simulink model "actuator_control"  (R2015a)
settings: Solver=FixedStepDiscrete  StartTime=0.0  StopTime=inf  FixedStep=sample_time  RelTol=1e-3
undefined symbols (not defined in the file): A_kalman_swing_load, A_lpf_dtau, B1_lpf_dtau, B2_lpf_dtau, B_kalman_swing_load, C_kalman_swing_load, Discrete, fdesignblkfcn, gcbh, initial_dx_estimate, j_segments, k_sea_low, lateral_motor_efficiency, P0_kalman_swing_load, sample_time, swing_collision_damping_rate, Time
libraries: simulink x11, dsparch4 x6, ctrlSharedLib x4, dspfdesign x2
(part 1 of 2)
settings Model: CovSFcnEnable=off  Creator=wmartin  LastModifiedBy=wmartin
settings SolverCC: EnableConcurrentExecution=on
settings DataIOCC: MaxDataPoints=1000000000  SaveFormat=StructureWithTime  SaveOutput=off  DSMLogging=off  SaveTime=off
settings OptimizationCC: BlockReduction=off  OptimizeBlockIOStorage=off  BufferReuse=off  GlobalBufferReuse=off  ExpressionFolding=off  LocalBlockOutputs=off  SimCompilerOptimization=on
settings DebuggingCC: SolverPrmCheckMsg=warning
settings HardwareCC: ProdIntDivRoundTo=Zero  ProdEndianess=LittleEndian  ProdLongLongMode=on  ProdHWDeviceType=Generic->32-bit x86 compatible
settings ModelReferenceCC: UpdateModelReferenceTargets=AssumeUpToDate  ModelReferenceNumInstancesAllowed=Single  ModelReferenceMinAlgLoopOccurrences=on
settings RTWCC: SystemTargetFile=slrt.tlc  TemplateMakefile=slrt_default_tmf  Description=Simulink Real-Time  RTWVerbose=off  RTWCompilerOptimization=on
settings SimulinkRealTimeCC: GeneratePreprocessorConditionals=Disable all  ExtMode=off

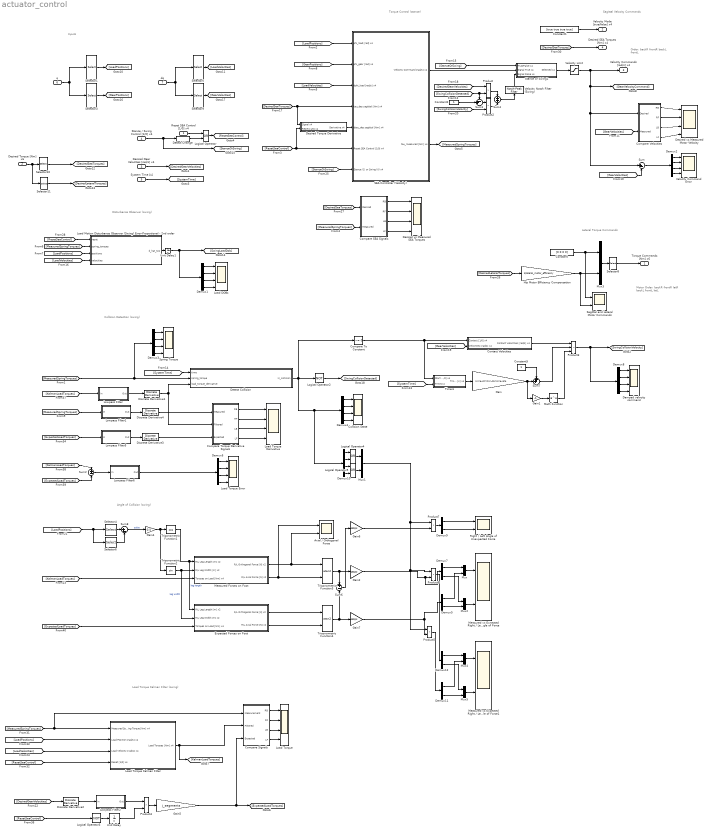
== system actuator_control ==
  note: Order:
      | backR
      | frontR
      | backL
      | frontL
  note: Motor Order:
      |
      | backR
      | frontR
      | latR
      | backL
      | frontL
      | latL
  note: Torque Control (stance)
  note: Inputs
  note: Disturbance Observer (swing)
  note: Lateral Torque Commands
  note: Sagittal Velocity Commands
  note: Collision Detection (swing)
  note: Load Torque Kalman Filter (swing)
  note: Angle of Collision (swing)
  Reset SEA Control [1/0] x4 : Inport  OutDataTypeStr=boolean  PortDimensions=4  SampleTime=sample_time
  Desired Torque [Nm] x6 : Inport  Port=2  OutDataTypeStr=double  PortDimensions=6  SampleTime=sample_time
  Desired Gear Velocities [rad/s] x4 : Inport  Port=3  OutDataTypeStr=double  PortDimensions=4  SampleTime=sample_time
  Stance / Swing Control [1/0] x4 : Inport  Port=4  OutDataTypeStr=boolean  PortDimensions=4  SampleTime=sample_time
  System Time [s] : Inport  Port=5  OutDataTypeStr=double  PortDimensions=1  SampleTime=sample_time
  q : Inport  Port=6  OutDataTypeStr=double  PortDimensions=13  SampleTime=sample_time
  dq : Inport  Port=7  OutDataTypeStr=double  PortDimensions=13  SampleTime=sample_time
  Axial / Orthogonal Force : Scope  NumInputPorts=2
      settings: YMin=-120~-175  YMax=120~150  SampleInput=on
  Collision State : Scope  NumInputPorts=4
      settings: YMin=0~-4~-1~-2.25  YMax=6~4~0.75~0  SaveName=LoadDOB_history2  SampleInput=on
  Compare To Constant : simulink/Logic and Bit Operations/Compare To Constant  relop=~=  const=0  OutDataTypeStr=boolean
  Compare SEA Signals : Subsystem
  Compare Signals : Subsystem
  Compare Torque Derivative Signals : Subsystem
  Compare Velocities : Subsystem
  Constant : Constant  Value=[0 0 0 0]
  Constant1 : Constant  Value=[true true true true]
  Constant2 : Constant
  Constant5 : Constant
  Contact Velocities : Subsystem
  Damped velocity command : Scope  NumInputPorts=4
      settings: YMin=0~-4~-1~-2.25  YMax=6~4~0.75~0  SaveName=LoadDOB_history6  SampleInput=on
  Demux{1..4,6,8,10} (7 alike) : Demux
  Demux{5,7,9,11..12} (5 alike) : Demux  Outputs=2
  Desired Torque Derivative : Subsystem
  Desired vs Measured Motor Velocity : Scope  NumInputPorts=4
      settings: YMin=-0.03~-0.03~-0.025~-0.025  YMax=0.02~0.025~0.02~0.02  SaveName=ScopeData14  SampleInput=on
  Desired vs Measured SEA Torques : Scope  NumInputPorts=4
      settings: YMin=-35~-75~-500~-200  YMax=50~75~150~550  SaveName=SeaTorques  SampleInput=on  SampleTime=sample_time
  Detect Change : simulink/Logic and Bit Operations/Detect Change  vinit=0  InputProcessing=Inherited  OutDataTypeStr=boolean
  Detect Collision : MATLAB Function  TreatAsAtomicUnit=on
  Discrete Derivative{1..4} (4 alike) : simulink/Discrete/Discrete Derivative  gainval=1.0  ICPrevScaledInput=0.0  OutMin=[]  OutMax=[]  OutDataType=fixdt(1, 16)  OutScaling=2^-10  DoSatur=off
  Expected Forces on Foot : Subsystem
  Gain : Gain  Gain=swing_collision_damping_rate
  Gain1 : Gain  Gain=-1
  Gain2 : Gain  Gain=180/pi
  Gain4 : Gain  Gain=0.5
  Gain5 : Gain  Gain=j_segments
  Gain6 : Gain  Gain=180/pi
  Gain7 : Gain  Gain=180/pi
  Hip Motor Efficiency Compensation : Gain  Gain=1/lateral_motor_efficiency
  Load DOBs : Scope  NumInputPorts=4
      settings: YMin=-12~-7~2.7~-0.5  YMax=-8.75~1~4.1~2  SaveName=LoadDOB_history  SampleInput=on
  Load Motion Disturbance Observer (Swing) Error-Proportional - 2nd order : MATLAB Function  TreatAsAtomicUnit=on
  Load Torque : Scope  NumInputPorts=4
      settings: TimeRange=34.366  YMin=-300~-400~-100~-200  YMax=100~150~400~800  SaveName=LoadDOB_history3  SampleInput=on
  Load Torque Derivative : Scope  NumInputPorts=4
      settings: TimeRange=50.096  YMin=-4122.660296851378~-4185.660018993349~-3974.358974358969~-4680.851063829847  YMax=3871.203105284947~4522.792022792026~4743.58974358975~5531.914893616988  SaveName=LoadDOB_history4  SampleInput=on
  Load Torque Error : Scope  NumInputPorts=4
      settings: YMin=-100~-125~-125~-125  YMax=125~100~125~100  SaveName=LoadDOB_history5  SampleInput=on
  Load Torque Kalman Filter : Subsystem
  Logical Operator : Logic  Operator=OR  AllPortsSameDT=off  OutDataTypeStr=boolean
  Logical Operator2 : Logic  Operator=NOT  AllPortsSameDT=off  OutDataTypeStr=boolean
  Logical Operator3 : Logic  Operator=NOT  AllPortsSameDT=off  OutDataTypeStr=boolean
  Logical Operator4 : Logic  Operator=OR  AllPortsSameDT=off  OutDataTypeStr=boolean
  Logical Operator5 : Logic  Operator=OR  AllPortsSameDT=off  OutDataTypeStr=boolean
  Lowpass Filter : Subsystem  DialogController=fdesignblkfcn  InitFcn=fdesignblkfcn(gcbh, {'InitFcn'});  mask(Lowpass Filter){}
      mask help: Design a lowpass filter
      settings: CopyFcn=fdesignblkfcn(gcbh, {'CopyFcn'});
      mask Help: helpview(mapfilelocation('dsp'), 'dsplowpassfilter');
      mask Display: disp('Lowpass')
  Lowpass Filter1 : Subsystem  DialogController=fdesignblkfcn  InitFcn=fdesignblkfcn(gcbh, {'InitFcn'});  mask(Lowpass Filter){}
      mask help: Design a lowpass filter
      settings: CopyFcn=fdesignblkfcn(gcbh, {'CopyFcn'});
      mask Help: helpview(mapfilelocation('dsp'), 'dsplowpassfilter');
      mask Display: disp('Lowpass')
  Lowpass Filter2 : Subsystem  DialogController=fdesignblkfcn  InitFcn=fdesignblkfcn(gcbh, {'InitFcn'});  mask(Lowpass Filter){}
      mask help: Design a lowpass filter
      settings: CopyFcn=fdesignblkfcn(gcbh, {'CopyFcn'});
      mask Help: helpview(mapfilelocation('dsp'), 'dsplowpassfilter');
      mask Display: disp('Lowpass')
  Lowpass Filter5 : Subsystem  DialogController=fdesignblkfcn  InitFcn=fdesignblkfcn(gcbh, {'InitFcn'});  mask(Lowpass Filter){}
      mask help: Design a lowpass filter
      settings: CopyFcn=fdesignblkfcn(gcbh, {'CopyFcn'});
      mask Help: helpview(mapfilelocation('dsp'), 'dsplowpassfilter');
      mask Display: disp('Lowpass')
  Lowpass Filter6 : Subsystem  DialogController=fdesignblkfcn  InitFcn=fdesignblkfcn(gcbh, {'InitFcn'});  mask(Lowpass Filter){}
      mask help: Design a lowpass filter
      settings: CopyFcn=fdesignblkfcn(gcbh, {'CopyFcn'});
      mask Help: helpview(mapfilelocation('dsp'), 'dsplowpassfilter');
      mask Display: disp('Lowpass')
  Math Function : Math  SaturateOnIntegerOverflow=on
  Measured Forces on Foot : Subsystem
  Measured vs Expected Right / Left Angle of Force : Scope  NumInputPorts=2
      settings: TimeRange=45  YMin=-200~-200  YMax=200~200  SampleInput=on
  Measured vs Expected Right / Left Angle of Force1 : Scope  NumInputPorts=2
      settings: TimeRange=45  YMin=-1~-200  YMax=1~200  SaveName=ScopeData8  SampleInput=on
  Mux{,1..5} (6 alike) : Mux  Inputs=2
  Product{,2,4..7} (6 alike) : Product
  Product3 : Product  Inputs=3
  Right / Left Angle of Unexpected Force : Scope  NumInputPorts=2
      settings: TimeRange=45  YMin=-350~-400  YMax=300~350  SaveName=ScopeData3  SampleInput=on
  SEA Controller (Velocity) : Subsystem
  Sagittal and Lateral Motor Commands : Scope  NumInputPorts=2
      settings: YMin=-1~0  YMax=1~65  SaveName=ScopeData2  SampleInput=on
  Selector1 : Selector  InputPortWidth=13  Indices=[1 3 5 7]
  Selector10 : Selector  InputPortWidth=6  Indices=[1 2 4 5]
  Selector11 : Selector  InputPortWidth=6  Indices=[3 6]
  Selector3 : Selector  InputPortWidth=13  Indices=[2 4 6 8]
  Selector4 : Selector  InputPortWidth=4  Indices=[1 3]
  Selector5 : Selector  InputPortWidth=13  Indices=[1 3 5 7]
  Selector6 : Selector  InputPortWidth=4  Indices=[2 4]
  Selector8 : Selector  InputPortWidth=6  Indices=[1 2 5 3 4 6]
  Selector9 : Selector  InputPortWidth=13  Indices=[2 4 6 8]
  Spring Torque : Scope  NumInputPorts=4
      settings: YMin=-75~-75~-75~-75  YMax=75~75~75~75  SaveName=LoadDOB_history1  SampleInput=on
  Stance or Swing1 : Subsystem
  Sum : Sum  Inputs=|+-
  Sum2 : Sum  Inputs=+|-
  Sum3 : Sum  Inputs=-+|
  Sum4 : Sum  Inputs=+|+
  Sum6 : Sum  Inputs=+|-
  Sum7 : Sum  Inputs=++|
  Sum8 : Sum  Inputs=|+-
  Timers : Subsystem
  Trigonometric Function1 : Trigonometry  Operator=cos
  Trigonometric Function2 : Trigonometry
  Trigonometric Function3 : Trigonometry  Operator=atan2
  Trigonometric Function4 : Trigonometry  Operator=atan2
  Unit Delay : UnitDelay  SampleTime=-1
  Unit Delay1 : UnitDelay  SampleTime=sample_time
  Velocity Command Error : Scope  NumInputPorts=4
      settings: YMin=-0.5~-0.4~-0.5~-1.5  YMax=1.5~0.5~0.9~0.75  SaveName=ScopeData6  SampleInput=on
  Velocity Limit : Saturate  UpperLimit=8  LowerLimit=-8
      settings: AttributesFormatString=Hi: %<UpperLimit>\nLo: %<LowerLimit>
  Velocity Notch Filter (Swing) : dspfdesign/Notch-Peak Filter  Specification=Quality factor and center frequency  Bandwidth=27  QualityFactor=2.5  CenterFrequency=27  BandwidthCoefficient=0.72654  CenterFrequencyCoefficient=0  Output=Notch  InheritSampleRate=off  SampleRate=update_freq  SimulateUsing=Code generation
  Torque Commands [Nm] x6 : Outport  OutDataTypeStr=double  PortDimensions=6  SampleTime=sample_time  InitialOutput=[0 0 0 0 0 0]
  Velocity Mode [true/false] x4 : Outport  Port=2  InitialOutput=[false false false false]
  Velocity Commands [rad/s] x4 : Outport  Port=3  InitialOutput=[0 0 0 0]
  Desired SEA Torques [Nm] x4 : Outport  Port=4  InitialOutput=[false false false false]
  wires:
  SEA Controller (Velocity)/2(tau_measured [Nm] x4) -> [MeasuredSpringTorques]
  Selector8/1 -> Torque Commands [Nm] x6/1
  q/1 -> Selector1/1, Selector3/1
  [LoadPositions] -> SEA Controller (Velocity)/1(phi_load [rad] x4)
  [DesiredSeaTorques] -> Desired Torque Derivative/1(Signal x4), SEA Controller (Velocity)/4(tau_des sagittal [Nm] x4)
  [DesiredLateralTorques] -> Hip Motor Efficiency Compensation/1
  Mux3/1 -> Selector8/1
  Desired Torque Derivative/1(Derivative x4) -> SEA Controller (Velocity)/5(dtau_des sagittal [Nm] x4)
  Constant/1 -> Sagittal and Lateral Motor Commands/1, Mux3/1
  Hip Motor Efficiency Compensation/1 -> Sagittal and Lateral Motor Commands/2, Mux3/2
  Compare SEA Signals/1(RB) -> Desired vs Measured SEA Torques/1
  Compare SEA Signals/2(RF) -> Desired vs Measured SEA Torques/2
  Compare SEA Signals/3(LB) -> Desired vs Measured SEA Torques/3
  Compare SEA Signals/4(LF) -> Desired vs Measured SEA Torques/4
  Compare Velocities/4(LF) -> Desired vs Measured Motor Velocity/4
  Compare Velocities/3(LB) -> Desired vs Measured Motor Velocity/3
  Compare Velocities/1(RB) -> Desired vs Measured Motor Velocity/1
  Compare Velocities/2(RF) -> Desired vs Measured Motor Velocity/2
  Load Motion Disturbance Observer (Swing) Error-Proportional - 2nd order/1(d_hat_tp1) -> Unit Delay1/1
  [MeasuredSpringTorques] -> Compare SEA Signals/2(Measured)
  [MeasuredSpringTorques] -> Load Motion Disturbance Observer (Swing) Error-Proportional - 2nd order/2(spring_torques)
  Selector1/1 -> [LoadPositions]
  Selector5/1 -> [LoadVelocities]
  [LoadPositions] -> Load Motion Disturbance Observer (Swing) Error-Proportional - 2nd order/3(positions)
  [LoadVelocities] -> Load Motion Disturbance Observer (Swing) Error-Proportional - 2nd order/4(velocities)
  Desired Torque [Nm] x6/1 -> Selector11/1, Selector10/1
  Selector11/1 -> [DesiredLateralTorques]
  [DesiredSeaTorques] -> Compare SEA Signals/1(Desired)
  [ResetSeaControl] -> Desired Torque Derivative/2(Reset [1/0] x4), SEA Controller (Velocity)/6(Reset SEA Control [1/0] x4)
  [ResetSeaControl] -> Load Motion Disturbance Observer (Swing) Error-Proportional - 2nd order/1(reset)
  Constant1/1 -> Velocity Mode [true/false] x4/1
  Demux1/1 -> Load DOBs/1
  Demux1/2 -> Load DOBs/2
  Demux1/3 -> Load DOBs/3
  Demux1/4 -> Load DOBs/4
  Unit Delay1/1 -> [SwingLoadDob], Demux1/1
  Stance / Swing Control [1/0] x4/1 -> [StanceOrSwing], Detect Change/1
  [StanceOrSwing] -> SEA Controller (Velocity)/7(Stance (1) or Swing (0) x4)
  Logical Operator/1 -> [ResetSeaControl]
  Reset SEA Control [1/0] x4/1 -> Logical Operator/1
  [DesiredSeaTorques] -> Desired SEA Torques [Nm] x4/1
  [LoadVelocities] -> SEA Controller (Velocity)/3(dphi_load [rad/s] x4)
  Selector3/1 -> [GearPositions]
  dq/1 -> Selector5/1, Selector9/1
  [GearPositions] -> SEA Controller (Velocity)/2(phi_gear [rad] x4)
  [GearVelocities] -> Compare Velocities/2(Measured)
  [GearVelocities] -> Sum/2
  Sum/1 -> Demux2/1
  [DesiredGearVelocities] -> Product/1
  Demux2/4 -> Velocity Command Error/4
  Demux2/3 -> Velocity Command Error/3
  Demux2/2 -> Velocity Command Error/2
  Demux2/1 -> Velocity Command Error/1
  Demux3/4 -> Spring Torque/4
  Demux3/3 -> Spring Torque/3
  Demux3/2 -> Spring Torque/2
  Demux3/1 -> Spring Torque/1
  [SwingCollisionDetected] -> Sum3/1, Product/2
  Selector10/1 -> [DesiredSeaTorques]
  Constant2/1 -> Sum3/2
  [SwingCollisionVelocity] -> Product2/2
  Product/1 -> Sum4/1
  Product2/1 -> Sum4/2
  Sum3/1 -> Product2/1
  [KalmanLoadTorques] -> Lowpass Filter/1(In)
  Detect Collision/1(in_collision) -> Compare To Constant/1, Demux10/1, Demux4/1, Logical Operator2/1
  Stance or Swing1/1(Selected x4) -> Velocity Limit/1
  SEA Controller (Velocity)/1(Velocity Command [rad/s] x4) -> Stance or Swing1/2(Signal True x4)
  [StanceOrSwing] -> Stance or Swing1/1(True/False x4)
  Detect Change/1 -> Logical Operator/2
  Desired Gear Velocities [rad/s] x4/1 -> [DesiredGearVelocities]
  [GearVelocities] -> Contact Velocities/2(Velocities [rad/s] x4)
  Contact Velocities/1(Contact Velocities [rad/s] x4) -> Product3/1
  Compare To Constant/1 -> Contact Velocities/1(Contact [1/0] x4), Timers/1(Start [1/0] x4)
  Timers/1(Timer [s] x4) -> Gain/1
  Gain/1 -> Gain1/1, Sum7/2
  Constant5/1 -> Sum7/1
  Gain1/1 -> Math Function/1
  Math Function/1 -> Product3/3
  Product3/1 -> [SwingCollisionVelocity], Demux8/1
  Demux8/3 -> Damped velocity command/3
  Demux8/2 -> Damped velocity command/2
  Demux8/1 -> Damped velocity command/1
  Demux8/4 -> Damped velocity command/4
  [SystemTime] -> Timers/2(Time [s])
  Sum4/1 -> Velocity Notch Filter (Swing)/1
  Selector9/1 -> [GearVelocities]
  System Time [s]/1 -> [SystemTime]
  [SystemTime] -> Detect Collision/1(time)
  Demux4/3 -> Collision State/3
  Demux4/2 -> Collision State/2
  Demux4/1 -> Collision State/1
  Demux4/4 -> Collision State/4
  Logical Operator2/1 -> [SwingCollisionDetected]
  Selector4/1 -> Sum8/1
  Sum8/1 -> Gain4/1  "splay"
  Gain4/1 -> Trigonometric Function2/1, Trigonometric Function1/1
  [LoadPositions] -> Selector6/1, Selector4/1
  Demux7/2 -> Mux2/1
  Demux7/1 -> Mux/1
  [LoadVelocities] -> Load Torque Kalman Filter/3(Load Velocity [rad/s] x4)
  [ResetSeaControl] -> Load Torque Kalman Filter/4(Reset [1/0] x4)
  Compare Signals/3(LB) -> Load Torque/3
  Compare Signals/2(RF) -> Load Torque/2
  Compare Signals/4(LF) -> Load Torque/4
  Compare Signals/1(RB) -> Load Torque/1
  Load Torque Kalman Filter/1(Load Torques [Nm] x4) -> [KalmanLoadTorques], Compare Signals/2(Filtered)
  [MeasuredSpringTorques] -> Compare Signals/1(Measurement), Load Torque Kalman Filter/1(Measured Spring Torque [Nm] x4)
  [LoadPositions] -> Load Torque Kalman Filter/2(Load Position [rad/s] x4)
  Trigonometric Function3/1 -> Sum6/1, Gain2/1
  Product4/1 -> Gain5/1
  Gain5/1 -> [ExpectedLoadTorques], Compare Signals/3(Expected)
  Discrete Derivative2/1 -> Lowpass Filter2/1(In)
  Logical Operator3/1 -> Unit Delay/1
  [ResetSeaControl] -> Logical Operator3/1
  Unit Delay/1 -> Product4/2
  [ExpectedLoadTorques] -> Lowpass Filter5/1(In)
  Lowpass Filter5/1(Out) -> Discrete Derivative3/1
  Compare Torque Derivative Signals/4(LF) -> Load Torque Derivative/4
  Compare Torque Derivative Signals/3(LB) -> Load Torque Derivative/3
  Compare Torque Derivative Signals/2(RF) -> Load Torque Derivative/2
  Compare Torque Derivative Signals/1(RB) -> Load Torque Derivative/1
  [MeasuredSpringTorques] -> Lowpass Filter1/1(In)
  Lowpass Filter1/1(Out) -> Discrete Derivative4/1
  Discrete Derivative4/1 -> Compare Torque Derivative Signals/1(Measured)
  Demux6/3 -> Load Torque Error/3
  Demux6/2 -> Load Torque Error/2
  Demux6/1 -> Load Torque Error/1
  Demux6/4 -> Load Torque Error/4
  [KalmanLoadTorques] -> Sum2/1
  [ExpectedLoadTorques] -> Sum2/2
  Sum2/1 -> Lowpass Filter6/1(In)
  [DesiredGearVelocities] -> Discrete Derivative2/1
  Discrete Derivative3/1 -> Compare Torque Derivative Signals/3(Expected)
  Selector6/1 -> Sum8/2
  Demux5/2 -> Mux2/2
  Demux5/1 -> Mux/2
  Demux10/1 -> Logical Operator4/1
  Demux10/2 -> Logical Operator4/2
  Demux10/4 -> Logical Operator5/2
  Demux10/3 -> Logical Operator5/1
  Logical Operator4/1 -> Mux1/1
  Logical Operator5/1 -> Mux1/2
  Sum7/1 -> Product3/2
  Discrete Derivative1/1 -> Compare Torque Derivative Signals/2(Filtered), Detect Collision/3(load_torque_derivative)
  Lowpass Filter6/1(Out) -> Demux6/1
  Lowpass Filter/1(Out) -> Discrete Derivative1/1
  Lowpass Filter2/1(Out) -> Product4/1
  Trigonometric Function1/1 -> Expected Forces on Foot/1(R/L Leg Length [m] x2), Measured Forces on Foot/1(R/L Leg Length [m] x2)  "leg length"
  Trigonometric Function2/1 -> Measured Forces on Foot/2(R/L Leg Width [m] x2), Expected Forces on Foot/2(R/L Leg Width [m] x2)  "leg width"
  [KalmanLoadTorques] -> Measured Forces on Foot/3(Torques on Load [Nm] x4)
  Measured Forces on Foot/1(R/L Orthogonal Force [N] x2) -> Trigonometric Function3/1, Axial / Orthogonal Force/2
  Measured Forces on Foot/2(R/L Axial Force [N] x2) -> Axial / Orthogonal Force/1, Trigonometric Function3/2
  [ExpectedLoadTorques] -> Expected Forces on Foot/3(Torques on Load [Nm] x4)
  Expected Forces on Foot/1(R/L Orthogonal Force [N] x2) -> Trigonometric Function4/1
  Trigonometric Function4/1 -> Sum6/2, Gain7/1
  Gain6/1 -> Product7/2
  Demux9/1 -> Right / Left Angle of Unexpected Force/1
  Demux9/2 -> Right / Left Angle of Unexpected Force/2
  Expected Forces on Foot/2(R/L Axial Force [N] x2) -> Trigonometric Function4/2
  Mux2/1 -> Measured vs Expected Right / Left Angle of Force/2
  Mux/1 -> Measured vs Expected Right / Left Angle of Force/1
  Gain7/1 -> Demux5/1, Product5/2
  Gain2/1 -> Demux7/1, Product6/2
  Mux1/1 -> Product7/1, Product5/1, Product6/1
  Sum6/1 -> Gain6/1
  Product7/1 -> Demux9/1
  Demux12/2 -> Mux5/1
  Demux12/1 -> Mux4/1
  Demux11/2 -> Mux5/2
  Demux11/1 -> Mux4/2
  Mux5/1 -> Measured vs Expected Right / Left Angle of Force1/2
  Mux4/1 -> Measured vs Expected Right / Left Angle of Force1/1
  Product6/1 -> Demux12/1
  Product5/1 -> Demux11/1
  Velocity Notch Filter (Swing)/1 -> Stance or Swing1/3(Signal False x4)
  Velocity Limit/1 -> [GearVelocityCommand], Sum/1, Compare Velocities/1(Desired), Velocity Commands [rad/s] x4/1
  [MeasuredSpringTorques] -> Demux3/1, Detect Collision/2(spring_torque)

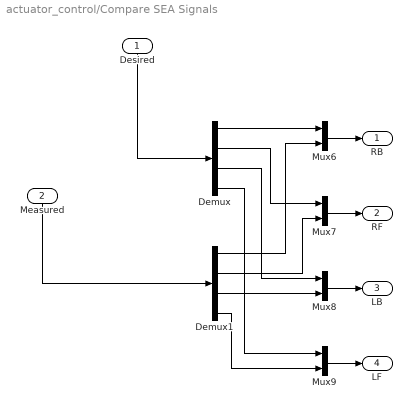
== system actuator_control/Compare SEA Signals ==
  Desired : Inport
  Measured : Inport  Port=2
  Demux : Demux
  Demux1 : Demux
  Mux{6..9} (4 alike) : Mux  Inputs=2
  RB : Outport
  RF : Outport  Port=2
  LB : Outport  Port=3
  LF : Outport  Port=4
  wires:
  Demux/3 -> Mux8/1
  Demux/2 -> Mux7/1
  Demux1/1 -> Mux6/2
  Demux/1 -> Mux6/1
  Demux/4 -> Mux9/1
  Demux1/4 -> Mux9/2
  Measured/1 -> Demux1/1
  Demux1/2 -> Mux7/2
  Desired/1 -> Demux/1
  Demux1/3 -> Mux8/2
  Mux6/1 -> RB/1
  Mux7/1 -> RF/1
  Mux9/1 -> LF/1
  Mux8/1 -> LB/1

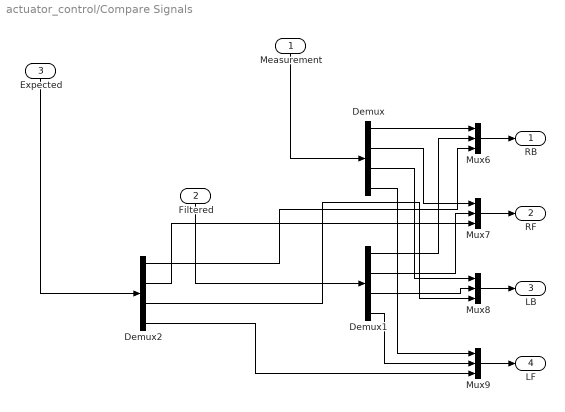
== system actuator_control/Compare Signals ==
  Measurement : Inport
  Filtered : Inport  Port=2
  Expected : Inport  Port=3
  Demux : Demux
  Demux1 : Demux
  Demux2 : Demux
  Mux{6..9} (4 alike) : Mux  Inputs=3
  RB : Outport
  RF : Outport  Port=2
  LB : Outport  Port=3
  LF : Outport  Port=4
  wires:
  Mux8/1 -> LB/1
  Mux9/1 -> LF/1
  Mux7/1 -> RF/1
  Mux6/1 -> RB/1
  Demux1/3 -> Mux8/2
  Measurement/1 -> Demux/1
  Demux1/2 -> Mux7/2
  Filtered/1 -> Demux1/1
  Demux1/4 -> Mux9/2
  Demux/4 -> Mux9/1
  Demux/1 -> Mux6/1
  Demux1/1 -> Mux6/2
  Demux/2 -> Mux7/1
  Demux/3 -> Mux8/1
  Expected/1 -> Demux2/1
  Demux2/1 -> Mux6/3
  Demux2/2 -> Mux7/3
  Demux2/3 -> Mux8/3
  Demux2/4 -> Mux9/3

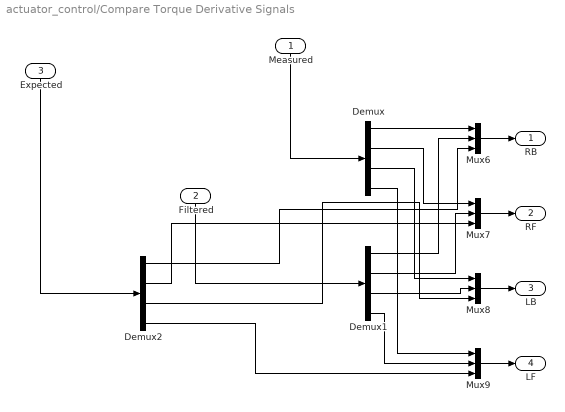
== system actuator_control/Compare Torque Derivative Signals ==
  Measured : Inport
  Filtered : Inport  Port=2
  Expected : Inport  Port=3
  Demux : Demux
  Demux1 : Demux
  Demux2 : Demux
  Mux{6..9} (4 alike) : Mux  Inputs=3
  RB : Outport
  RF : Outport  Port=2
  LB : Outport  Port=3
  LF : Outport  Port=4
  wires:
  Demux2/4 -> Mux9/3
  Demux2/3 -> Mux8/3
  Demux2/2 -> Mux7/3
  Demux2/1 -> Mux6/3
  Expected/1 -> Demux2/1
  Demux/3 -> Mux8/1
  Demux/2 -> Mux7/1
  Demux1/1 -> Mux6/2
  Demux/1 -> Mux6/1
  Demux/4 -> Mux9/1
  Demux1/4 -> Mux9/2
  Filtered/1 -> Demux1/1
  Demux1/2 -> Mux7/2
  Measured/1 -> Demux/1
  Demux1/3 -> Mux8/2
  Mux6/1 -> RB/1
  Mux7/1 -> RF/1
  Mux9/1 -> LF/1
  Mux8/1 -> LB/1

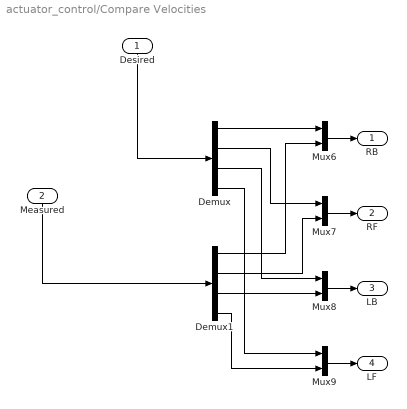
== system actuator_control/Compare Velocities ==
  Desired : Inport
  Measured : Inport  Port=2
  Demux : Demux
  Demux1 : Demux
  Mux{6..9} (4 alike) : Mux  Inputs=2
  RB : Outport
  RF : Outport  Port=2
  LB : Outport  Port=3
  LF : Outport  Port=4
  wires:
  Demux1/3 -> Mux8/2
  Desired/1 -> Demux/1
  Demux1/2 -> Mux7/2
  Measured/1 -> Demux1/1
  Demux1/4 -> Mux9/2
  Demux/4 -> Mux9/1
  Demux/1 -> Mux6/1
  Demux1/1 -> Mux6/2
  Demux/2 -> Mux7/1
  Demux/3 -> Mux8/1
  Mux6/1 -> RB/1
  Mux7/1 -> RF/1
  Mux8/1 -> LB/1
  Mux9/1 -> LF/1

== system actuator_control/Contact Velocities ==
  Contact [1/0] x4 : Inport
  Velocities [rad/s] x4 : Inport  Port=2
  Demux : Demux
  Demux1 : Demux
  Mux : Mux
  Velocity on Contact : Subsystem
  Velocity on Contact1 : Subsystem
  Velocity on Contact2 : Subsystem
  Velocity on Contact3 : Subsystem
  Contact Velocities [rad/s] x4 : Outport
  wires:
  Mux/1 -> Contact Velocities [rad/s] x4/1
  Demux/2 -> Velocity on Contact1/Trigger
  Velocity on Contact/1(out) -> Mux/1
  Contact [1/0] x4/1 -> Demux/1
  Velocity on Contact1/1(out) -> Mux/2
  Demux/3 -> Velocity on Contact2/Trigger
  Demux/4 -> Velocity on Contact3/Trigger
  Demux/1 -> Velocity on Contact/Trigger
  Velocity on Contact3/1(out) -> Mux/4
  Velocity on Contact2/1(out) -> Mux/3
  Velocities [rad/s] x4/1 -> Demux1/1
  Demux1/1 -> Velocity on Contact/1(in)
  Demux1/2 -> Velocity on Contact1/1(in)
  Demux1/3 -> Velocity on Contact2/1(in)
  Demux1/4 -> Velocity on Contact3/1(in)

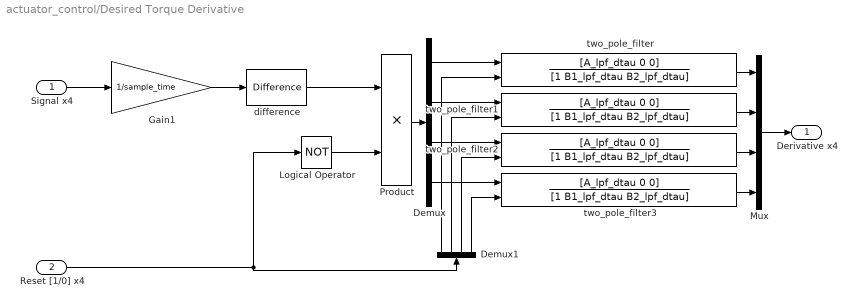
== system actuator_control/Desired Torque Derivative ==
  Signal x4 : Inport
  Reset [1/0] x4 : Inport  Port=2
  Demux : Demux
  Demux1 : Demux
  Gain1 : Gain  Gain=1/sample_time
  Logical Operator : Logic  Operator=NOT  AllPortsSameDT=off  OutDataTypeStr=boolean
  Mux : Mux
  Product : Product
  difference : simulink/Discrete/Difference  ICPrevInput=0.0  InputProcessing=Inherited  OutMin=[]  OutMax=[]  OutDataType=fixdt(1, 16)  OutScaling=2^-10  DoSatur=off
  two_pole_filter{,1..3} (4 alike) : DiscreteTransferFcn  Numerator=[A_lpf_dtau 0 0]  Denominator=[1 B1_lpf_dtau B2_lpf_dtau]  ExternalReset=Rising  SampleTime=sample_time
      settings: InputPortMap=u0,r7
  Derivative x4 : Outport
  wires:
  Demux/1 -> two_pole_filter/1
  difference/1 -> Product/1
  Mux/1 -> Derivative x4/1
  Signal x4/1 -> Gain1/1
  Gain1/1 -> difference/1
  Logical Operator/1 -> Product/2
  Reset [1/0] x4/1 -> Demux1/1, Logical Operator/1
  two_pole_filter/1 -> Mux/1
  Product/1 -> Demux/1
  two_pole_filter1/1 -> Mux/2
  two_pole_filter2/1 -> Mux/3
  two_pole_filter3/1 -> Mux/4
  Demux/2 -> two_pole_filter1/1
  Demux/3 -> two_pole_filter2/1
  Demux/4 -> two_pole_filter3/1
  Demux1/1 -> two_pole_filter/2
  Demux1/2 -> two_pole_filter1/2
  Demux1/3 -> two_pole_filter2/2
  Demux1/4 -> two_pole_filter3/2

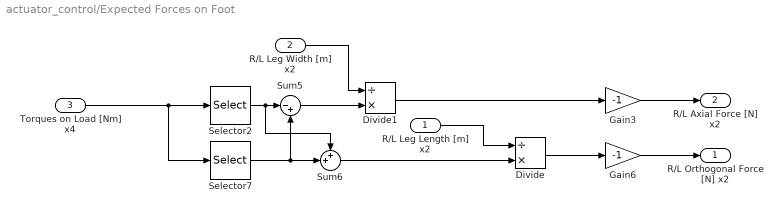
== system actuator_control/Expected Forces on Foot ==
  R/L Leg Length [m] x2 : Inport
  R/L Leg Width [m] x2 : Inport  Port=2
  Torques on Load [Nm] x4 : Inport  Port=3
  Divide : Product  Inputs=/*
  Divide1 : Product  Inputs=/*
  Gain3 : Gain  Gain=-1
  Gain6 : Gain  Gain=-1
  Selector2 : Selector  InputPortWidth=4  Indices=[1 3]
  Selector7 : Selector  InputPortWidth=4  Indices=[2 4]
  Sum5 : Sum  Inputs=|-+
  Sum6 : Sum  Inputs=++|
  R/L Orthogonal Force [N] x2 : Outport
  R/L Axial Force [N] x2 : Outport  Port=2
  wires:
  Gain6/1 -> R/L Orthogonal Force [N] x2/1
  Gain3/1 -> R/L Axial Force [N] x2/1
  Sum5/1 -> Divide1/2
  Selector7/1 -> Sum6/2, Sum5/2
  Sum6/1 -> Divide/2
  Selector2/1 -> Sum5/1, Sum6/1
  Divide1/1 -> Gain3/1
  Torques on Load [Nm] x4/1 -> Selector2/1, Selector7/1
  R/L Leg Width [m] x2/1 -> Divide1/1
  R/L Leg Length [m] x2/1 -> Divide/1
  Divide/1 -> Gain6/1

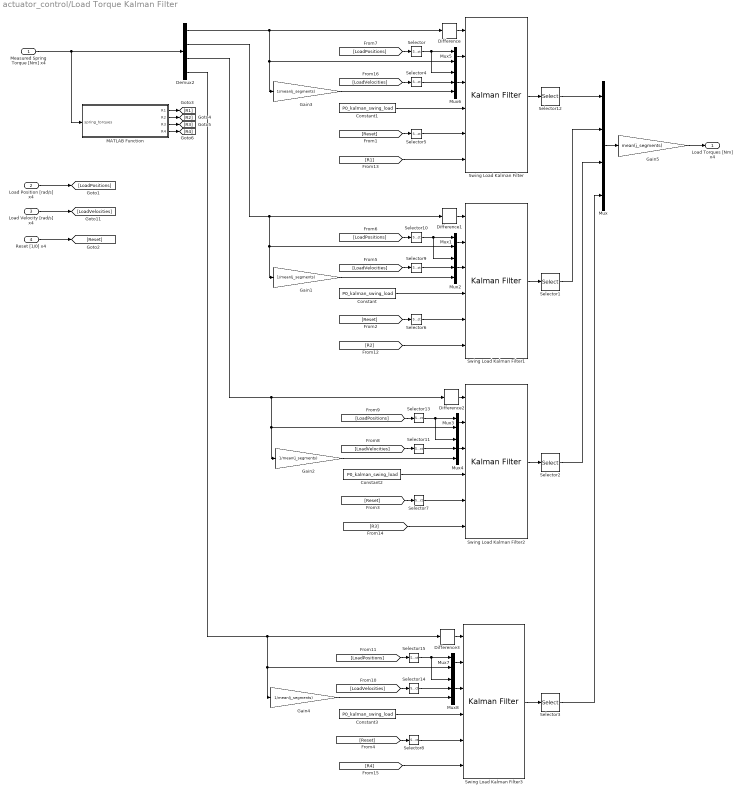
== system actuator_control/Load Torque Kalman Filter ==
  Measured Spring Torque [Nm] x4 : Inport
  Load Position [rad/s] x4 : Inport  Port=2
  Load Velocity [rad/s] x4 : Inport  Port=3
  Reset [1/0] x4 : Inport  Port=4
  Constant{,1..3} (4 alike) : Constant  Value=P0_kalman_swing_load
  Demux2 : Demux
  Difference{,1..3} (4 alike) : simulink/Discrete/Difference  ICPrevInput=0.0  InputProcessing=Inherited  OutMin=[]  OutMax=[]  OutDataType=fixdt(1, 16)  OutScaling=2^-10  DoSatur=off
  Gain{1..4} (4 alike) : Gain  Gain=1/mean(j_segments)
  Gain5 : Gain  Gain=mean(j_segments)
  MATLAB Function : MATLAB Function  TreatAsAtomicUnit=on
  Mux : Mux
  Mux{1,3,5,7} (4 alike) : Mux  Inputs=2
  Mux{2,4,6,8} (4 alike) : Mux  Inputs=3
  Selector : Selector  InputPortWidth=4  Indices=[1]
  Selector{1..3,12} (4 alike) : Selector  InputPortWidth=3  Indices=[3]
  Selector10 : Selector  InputPortWidth=4  Indices=[2]
  Selector11 : Selector  InputPortWidth=4  Indices=[3]
  Selector13 : Selector  InputPortWidth=4  Indices=[3]
  Selector14 : Selector  InputPortWidth=4  Indices=[4]
  Selector15 : Selector  InputPortWidth=4  Indices=[4]
  Selector4 : Selector  InputPortWidth=4  Indices=[1]
  Selector5 : Selector  InputPortWidth=4  Indices=[1]
  Selector6 : Selector  InputPortWidth=4  Indices=[2]
  Selector7 : Selector  InputPortWidth=4  Indices=[3]
  Selector8 : Selector  InputPortWidth=4  Indices=[4]
  Selector9 : Selector  InputPortWidth=4  Indices=[2]
  Swing Load Kalman Filter{,1..3} (4 alike) : ctrlSharedLib/Kalman Filter  TimeDomain=Discrete-Time  UseCurrentEstimator=on  ModelSource=Individual A, B, C, D matrices  ModelSourceVariable=A_kf  A=A_kalman_swing_load  B=B_kalman_swing_load  C=C_kalman_swing_load  D=0  NumberOfStates=2  NumberOfInputs=1  NumberOfOutputs=2  InitialEstimateSource=Input port  X0=initial_dx_estimate  P0=P0_kalman_transverse  UseK=off  UseGH=on  NumberOfProcessNoiseInputs=1  G=G_kalman_swing_load  TimeInvariantG=on  H=0  TimeInvariantH=on  Q=Q_kalman_SEA_torque_difference  TimeInvariantQ=on  R=1  TimeInvariantR=off  N=0  TimeInvariantN=on  AddInputPort=on  AddEnablePort=off  ExternalReset=Rising  OutputEstimatedY=off  OutputP=off  Ts=sample_time
  Load Torques [Nm] x4 : Outport
  wires:
  Mux6/1 -> Swing Load Kalman Filter/3
  Mux5/1 -> Swing Load Kalman Filter/2
  Difference/1 -> Swing Load Kalman Filter/1
  Demux2/1 -> Gain3/1, Mux5/2, Difference/1
  Swing Load Kalman Filter/1 -> Selector12/1
  Selector12/1 -> Mux/1
  Mux2/1 -> Swing Load Kalman Filter1/3
  Mux1/1 -> Swing Load Kalman Filter1/2
  Difference1/1 -> Swing Load Kalman Filter1/1
  Demux2/2 -> Gain1/1, Mux1/2, Difference1/1
  Gain1/1 -> Mux2/3
  Mux4/1 -> Swing Load Kalman Filter2/3
  Mux3/1 -> Swing Load Kalman Filter2/2
  Difference2/1 -> Swing Load Kalman Filter2/1
  Demux2/3 -> Difference2/1, Mux3/2, Gain2/1
  Gain2/1 -> Mux4/3
  Mux8/1 -> Swing Load Kalman Filter3/3
  Mux7/1 -> Swing Load Kalman Filter3/2
  Difference3/1 -> Swing Load Kalman Filter3/1
  Demux2/4 -> Difference3/1, Mux7/2, Gain4/1
  Gain4/1 -> Mux8/3
  Swing Load Kalman Filter1/1 -> Selector1/1
  Swing Load Kalman Filter3/1 -> Selector3/1
  Swing Load Kalman Filter2/1 -> Selector2/1
  Mux/1 -> Gain5/1
  Selector1/1 -> Mux/2
  Selector2/1 -> Mux/3
  Selector3/1 -> Mux/4
  Reset [1/0] x4/1 -> [Reset]
  Load Velocity [rad/s] x4/1 -> [LoadVelocities]
  Measured Spring Torque [Nm] x4/1 -> MATLAB Function/1(spring_torques), Demux2/1
  Gain5/1 -> Load Torques [Nm] x4/1
  Gain3/1 -> Mux6/3
  Load Position [rad/s] x4/1 -> [LoadPositions]
  [LoadPositions] -> Selector/1
  [LoadVelocities] -> Selector4/1
  Selector/1 -> Mux6/1, Mux5/1
  Selector4/1 -> Mux6/2
  [Reset] -> Selector5/1
  Selector5/1 -> Swing Load Kalman Filter/5
  [Reset] -> Selector6/1
  Selector6/1 -> Swing Load Kalman Filter1/5
  [Reset] -> Selector7/1
  Selector7/1 -> Swing Load Kalman Filter2/5
  [Reset] -> Selector8/1
  Selector8/1 -> Swing Load Kalman Filter3/5
  [LoadVelocities] -> Selector9/1
  [LoadPositions] -> Selector10/1
  [LoadVelocities] -> Selector11/1
  [LoadPositions] -> Selector13/1
  [LoadVelocities] -> Selector14/1
  [LoadPositions] -> Selector15/1
  Selector15/1 -> Mux8/1, Mux7/1
  Selector13/1 -> Mux4/1, Mux3/1
  Selector11/1 -> Mux4/2
  Selector14/1 -> Mux8/2
  Selector9/1 -> Mux2/2
  Selector10/1 -> Mux2/1, Mux1/1
  Constant/1 -> Swing Load Kalman Filter1/4
  MATLAB Function/1(R1) -> [R1]
  MATLAB Function/2(R2) -> [R2]
  MATLAB Function/3(R3) -> [R3]
  MATLAB Function/4(R4) -> [R4]
  [R2] -> Swing Load Kalman Filter1/6
  [R1] -> Swing Load Kalman Filter/6
  Constant1/1 -> Swing Load Kalman Filter/4
  [R3] -> Swing Load Kalman Filter2/6
  Constant2/1 -> Swing Load Kalman Filter2/4
  Constant3/1 -> Swing Load Kalman Filter3/4
  [R4] -> Swing Load Kalman Filter3/6

== system actuator_control/Lowpass Filter ==
  In : Inport
  Generated Filter Block : dsparch4/Biquad Filter  Tag=BlockMethodSubSystem  IIRFiltStruct=Direct form II  CoeffSource=Specify via dialog  BiQuadCoeffs=[1.0054190789171848 -2 1.0054190789171853 1 -1.9557970115108714 0.95685429506963915]  a0Flag=Warning  IC=0  ICnum=0  ICden=0  denAccumFracLength=30  denProdOutputFracLength=30  secondMemoryFracLength=15  roundingMode=Floor  overflowMode=off  ScaleValues=[0.0010519560093213882;92.733879468734756]  optimizeScaleValues=off  ScaleValueMode=Specify via input port (g)  scaleValueFracLength=14  FilterSource=Specify via dialog  FilterObject=Hm_biquad
  Out : Outport
  wires:
  Generated Filter Block/1 -> Out/1
  In/1 -> Generated Filter Block/1

== system actuator_control/Lowpass Filter1 ==
  In : Inport
  Generated Filter Block : dsparch4/Biquad Filter  Tag=BlockMethodSubSystem  IIRFiltStruct=Direct form II  CoeffSource=Specify via dialog  BiQuadCoeffs=[1.0054190789171848 -2 1.0054190789171853 1 -1.9557970115108714 0.95685429506963915]  a0Flag=Warning  IC=0  ICnum=0  ICden=0  denAccumFracLength=30  denProdOutputFracLength=30  secondMemoryFracLength=15  roundingMode=Floor  overflowMode=off  ScaleValues=[0.0010519560093213882;92.733879468734756]  optimizeScaleValues=off  ScaleValueMode=Specify via input port (g)  scaleValueFracLength=14  FilterSource=Specify via dialog  FilterObject=Hm_biquad
  Out : Outport
  wires:
  In/1 -> Generated Filter Block/1
  Generated Filter Block/1 -> Out/1

== system actuator_control/Lowpass Filter2 ==
  In : Inport
  Generated Filter Block : dsparch4/Biquad Filter  Tag=BlockMethodSubSystem  IIRFiltStruct=Direct form II  CoeffSource=Specify via dialog  BiQuadCoeffs=[0.42638734887522584 0.71004939850960869 0.42638734887522595 1 0.054295561672899631 0.19751119790393634]  a0Flag=Warning  IC=0  ICnum=0  ICden=0  denAccumFracLength=30  denProdOutputFracLength=30  secondMemoryFracLength=15  roundingMode=Floor  overflowMode=off  ScaleValues=[0.80099018345858064;1]  optimizeScaleValues=off  ScaleValueMode=Specify via input port (g)  scaleValueFracLength=14  FilterSource=Specify via dialog  FilterObject=Hm_biquad
  Out : Outport
  wires:
  In/1 -> Generated Filter Block/1
  Generated Filter Block/1 -> Out/1

== system actuator_control/Lowpass Filter5 ==
  In : Inport
  Generated Filter Block : dsparch4/Biquad Filter  Tag=BlockMethodSubSystem  IIRFiltStruct=Direct form II  CoeffSource=Specify via dialog  BiQuadCoeffs=[1.0054190789171848 -2 1.0054190789171853 1 -1.9557970115108714 0.95685429506963915]  a0Flag=Warning  IC=0  ICnum=0  ICden=0  denAccumFracLength=30  denProdOutputFracLength=30  secondMemoryFracLength=15  roundingMode=Floor  overflowMode=off  ScaleValues=[0.0010519560093213882;92.733879468734756]  optimizeScaleValues=off  ScaleValueMode=Specify via input port (g)  scaleValueFracLength=14  FilterSource=Specify via dialog  FilterObject=Hm_biquad
  Out : Outport
  wires:
  In/1 -> Generated Filter Block/1
  Generated Filter Block/1 -> Out/1

== system actuator_control/Lowpass Filter6 ==
  In : Inport
  Generated Filter Block : dsparch4/Biquad Filter  Tag=BlockMethodSubSystem  IIRFiltStruct=Direct form II  CoeffSource=Specify via dialog  BiQuadCoeffs=[1.0054190789171848 -2 1.0054190789171853 1 -1.9557970115108714 0.95685429506963915]  a0Flag=Warning  IC=0  ICnum=0  ICden=0  denAccumFracLength=30  denProdOutputFracLength=30  secondMemoryFracLength=15  roundingMode=Floor  overflowMode=off  ScaleValues=[0.0010519560093213882;92.733879468734756]  optimizeScaleValues=off  ScaleValueMode=Specify via input port (g)  scaleValueFracLength=14  FilterSource=Specify via dialog  FilterObject=Hm_biquad
  Out : Outport
  wires:
  Generated Filter Block/1 -> Out/1
  In/1 -> Generated Filter Block/1

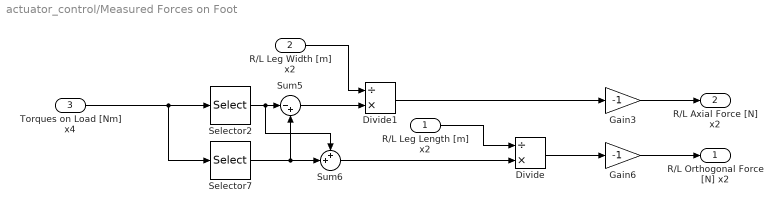
== system actuator_control/Measured Forces on Foot ==
  R/L Leg Length [m] x2 : Inport
  R/L Leg Width [m] x2 : Inport  Port=2
  Torques on Load [Nm] x4 : Inport  Port=3
  Divide : Product  Inputs=/*
  Divide1 : Product  Inputs=/*
  Gain3 : Gain  Gain=-1
  Gain6 : Gain  Gain=-1
  Selector2 : Selector  InputPortWidth=4  Indices=[1 3]
  Selector7 : Selector  InputPortWidth=4  Indices=[2 4]
  Sum5 : Sum  Inputs=|-+
  Sum6 : Sum  Inputs=++|
  R/L Orthogonal Force [N] x2 : Outport
  R/L Axial Force [N] x2 : Outport  Port=2
  wires:
  Divide/1 -> Gain6/1
  R/L Leg Length [m] x2/1 -> Divide/1
  R/L Leg Width [m] x2/1 -> Divide1/1
  Torques on Load [Nm] x4/1 -> Selector7/1, Selector2/1
  Divide1/1 -> Gain3/1
  Selector2/1 -> Sum6/1, Sum5/1
  Sum6/1 -> Divide/2
  Selector7/1 -> Sum5/2, Sum6/2
  Sum5/1 -> Divide1/2
  Gain3/1 -> R/L Axial Force [N] x2/1
  Gain6/1 -> R/L Orthogonal Force [N] x2/1

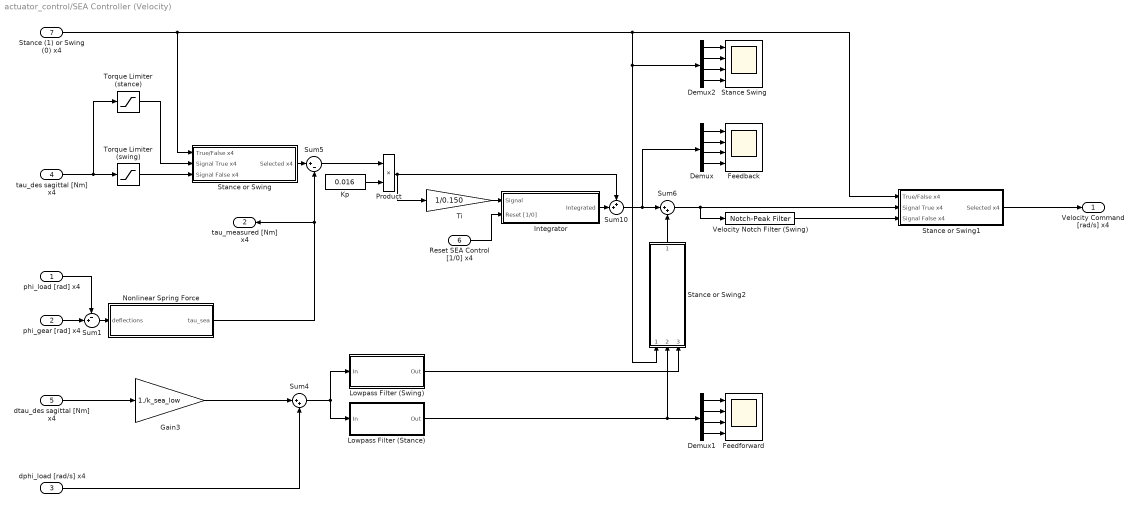
== system actuator_control/SEA Controller (Velocity) ==
  phi_load [rad] x4 : Inport
  phi_gear [rad] x4 : Inport  Port=2
  dphi_load [rad/s] x4 : Inport  Port=3
  tau_des sagittal [Nm] x4 : Inport  Port=4
  dtau_des sagittal [Nm] x4 : Inport  Port=5
  Reset SEA Control [1/0] x4 : Inport  Port=6
  Stance (1) or Swing (0) x4 : Inport  Port=7
  Demux : Demux
  Demux1 : Demux
  Demux2 : Demux
  Feedback : Scope  NumInputPorts=4
      settings: YMin=-4~-0.9~-5~-5  YMax=4.5~1~5~5  SaveName=ScopeData7  SampleInput=on
  Feedforward : Scope  NumInputPorts=4
      settings: YMin=-4~-0.9~-5~-5  YMax=4.5~1~5~5  SaveName=ScopeData4  SampleInput=on
  Gain3 : Gain  Gain=1./k_sea_low
  Integrator : Subsystem
  Kp : Constant  Value=0.016
  Lowpass Filter (Stance) : Subsystem  DialogController=fdesignblkfcn  InitFcn=fdesignblkfcn(gcbh, {'InitFcn'});  mask(Lowpass Filter){}
      mask help: Design a lowpass filter
      settings: CopyFcn=fdesignblkfcn(gcbh, {'CopyFcn'});
      mask Help: helpview(mapfilelocation('dsp'), 'dsplowpassfilter');
      mask Display: disp('Lowpass')
  Lowpass Filter (Swing) : Subsystem  DialogController=fdesignblkfcn  InitFcn=fdesignblkfcn(gcbh, {'InitFcn'});  mask(Lowpass Filter){}
      mask help: Design a lowpass filter
      settings: CopyFcn=fdesignblkfcn(gcbh, {'CopyFcn'});
      mask Help: helpview(mapfilelocation('dsp'), 'dsplowpassfilter');
      mask Display: disp('Lowpass')
  Nonlinear Spring Force : MATLAB Function  TreatAsAtomicUnit=on
  Product : Product
  Stance Swing : Scope  NumInputPorts=4
      settings: YMin=-4~-0.9~-5~-5  YMax=4.5~1~5~5  SaveName=ScopeData5  SampleInput=on
  Stance or Swing : Subsystem
  Stance or Swing1 : Subsystem
  Stance or Swing2 : Subsystem
  Sum1 : Sum  Inputs=-+|
  Sum10 : Sum  Inputs=++|
  Sum4 : Sum  Inputs=|++
  Sum5 : Sum  Inputs=|+-
  Sum6 : Sum  Inputs=|++
  Ti : Gain  Gain=1/0.150
  Torque Limiter (stance) : Saturate  UpperLimit=700  LowerLimit=-700
      settings: AttributesFormatString=Hi: %<UpperLimit>\nLo: %<LowerLimit>
  Torque Limiter (swing) : Saturate  UpperLimit=80  LowerLimit=-80
      settings: AttributesFormatString=Hi: %<UpperLimit>\nLo: %<LowerLimit>
  Velocity Notch Filter (Swing) : dspfdesign/Notch-Peak Filter  Specification=Quality factor and center frequency  Bandwidth=27  QualityFactor=2.5  CenterFrequency=27  BandwidthCoefficient=0.72654  CenterFrequencyCoefficient=0  Output=Notch  InheritSampleRate=off  SampleRate=update_freq  SimulateUsing=Code generation
  Velocity Command [rad/s] x4 : Outport  PortDimensions=4
  tau_measured [Nm] x4 : Outport  Port=2
  wires:
  Sum1/1 -> Nonlinear Spring Force/1(deflections)
  Nonlinear Spring Force/1(tau_sea) -> tau_measured [Nm] x4/1, Sum5/2
  Product/1 -> Ti/1, Sum10/1
  Sum6/1 -> Stance or Swing1/2(Signal True x4), Velocity Notch Filter (Swing)/1
  Gain3/1 -> Sum4/1
  dtau_des sagittal [Nm] x4/1 -> Gain3/1
  Reset SEA Control [1/0] x4/1 -> Integrator/2(Reset [1/0])
  Sum5/1 -> Product/1
  Integrator/1(Integrated) -> Sum10/2
  Ti/1 -> Integrator/1(Signal)
  dphi_load [rad/s] x4/1 -> Sum4/2
  Sum4/1 -> Lowpass Filter (Stance)/1(In), Lowpass Filter (Swing)/1(In)
  Lowpass Filter (Stance)/1(Out) -> Stance or Swing2/2(Signal True x4), Demux1/1
  Kp/1 -> Product/2
  Stance or Swing/1(Selected x4) -> Sum5/1
  Torque Limiter (swing)/1 -> Stance or Swing/3(Signal False x4)
  Torque Limiter (stance)/1 -> Stance or Swing/2(Signal True x4)
  Stance or Swing1/1(Selected x4) -> Velocity Command [rad/s] x4/1
  Velocity Notch Filter (Swing)/1 -> Stance or Swing1/3(Signal False x4)
  Demux/4 -> Feedback/4
  Demux/3 -> Feedback/3
  Demux/2 -> Feedback/2
  Demux/1 -> Feedback/1
  Demux1/1 -> Feedforward/1
  Demux1/2 -> Feedforward/2
  Demux1/3 -> Feedforward/3
  Demux1/4 -> Feedforward/4
  tau_des sagittal [Nm] x4/1 -> Torque Limiter (stance)/1, Torque Limiter (swing)/1
  phi_gear [rad] x4/1 -> Sum1/2
  phi_load [rad] x4/1 -> Sum1/1
  Stance (1) or Swing (0) x4/1 -> Demux2/1, Stance or Swing2/1(True/False x4), Stance or Swing1/1(True/False x4), Stance or Swing/1(True/False x4)
  Demux2/3 -> Stance Swing/3
  Demux2/2 -> Stance Swing/2
  Demux2/1 -> Stance Swing/1
  Demux2/4 -> Stance Swing/4
  Sum10/1 -> Demux/1, Sum6/1
  Lowpass Filter (Swing)/1(Out) -> Stance or Swing2/3(Signal False x4)
  Stance or Swing2/1(Selected x4) -> Sum6/2

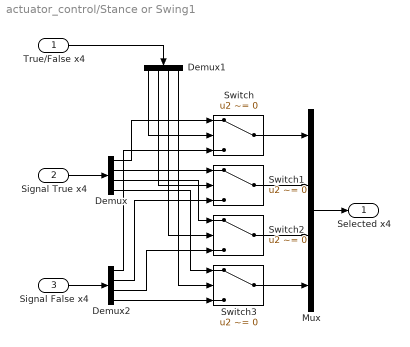
== system actuator_control/Stance or Swing1 ==
  True/False x4 : Inport
  Signal True x4 : Inport  Port=2
  Signal False x4 : Inport  Port=3
  Demux : Demux
  Demux1 : Demux
  Demux2 : Demux
  Mux : Mux
  Switch{,1..3} (4 alike) : Switch  Criteria=u2 ~= 0
  Selected x4 : Outport
  wires:
  Switch3/1 -> Mux/4
  Switch2/1 -> Mux/3
  Switch1/1 -> Mux/2
  Switch/1 -> Mux/1
  Demux1/4 -> Switch3/2
  Demux1/3 -> Switch2/2
  Demux1/2 -> Switch1/2
  Demux1/1 -> Switch/2
  Demux2/4 -> Switch3/3
  Demux2/3 -> Switch2/3
  Demux2/2 -> Switch1/3
  Demux2/1 -> Switch/3
  Demux/4 -> Switch3/1
  Demux/3 -> Switch2/1
  Demux/2 -> Switch1/1
  Demux/1 -> Switch/1
  Signal False x4/1 -> Demux2/1
  Signal True x4/1 -> Demux/1
  True/False x4/1 -> Demux1/1
  Mux/1 -> Selected x4/1

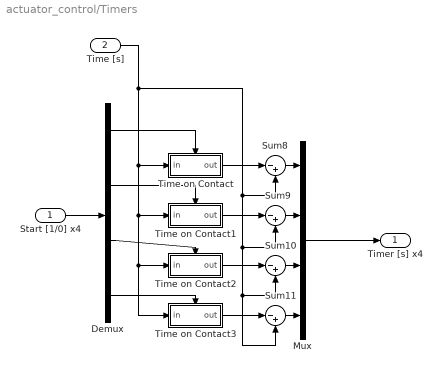
== system actuator_control/Timers ==
  Start [1/0] x4 : Inport
  Time [s] : Inport  Port=2
  Demux : Demux
  Mux : Mux
  Sum{8..11} (4 alike) : Sum  Inputs=|-+
  Time on Contact : Subsystem
  Time on Contact1 : Subsystem
  Time on Contact2 : Subsystem
  Time on Contact3 : Subsystem
  Timer [s] x4 : Outport
  wires:
  Sum10/1 -> Mux/3
  Sum11/1 -> Mux/4
  Demux/1 -> Time on Contact/Trigger
  Demux/4 -> Time on Contact3/Trigger
  Demux/3 -> Time on Contact2/Trigger
  Time on Contact3/1(out) -> Sum11/1
  Sum9/1 -> Mux/2
  Start [1/0] x4/1 -> Demux/1
  Sum8/1 -> Mux/1
  Time on Contact1/1(out) -> Sum9/1
  Demux/2 -> Time on Contact1/Trigger
  Time [s]/1 -> Time on Contact3/1(in), Time on Contact2/1(in), Time on Contact1/1(in), Time on Contact/1(in), Sum8/2, Sum9/2, Sum11/2, Sum10/2
  Mux/1 -> Timer [s] x4/1
  Time on Contact2/1(out) -> Sum10/1
  Time on Contact/1(out) -> Sum8/1

== system actuator_control/Contact Velocities/Velocity on Contact ==
  in : Inport
  Trigger : TriggerPort  ShowOutputPort=on  PortDimensions=1
  Subsystem : Subsystem
  out : Outport
  wires:
  Trigger/1 -> Subsystem/Enable
  Subsystem/1(out) -> out/1
  in/1 -> Subsystem/1(in)

== system actuator_control/Contact Velocities/Velocity on Contact1 ==
  in : Inport
  Trigger : TriggerPort  ShowOutputPort=on  PortDimensions=1
  Subsystem : Subsystem
  out : Outport
  wires:
  in/1 -> Subsystem/1(in)
  Subsystem/1(out) -> out/1
  Trigger/1 -> Subsystem/Enable

== system actuator_control/Contact Velocities/Velocity on Contact2 ==
  in : Inport
  Trigger : TriggerPort  ShowOutputPort=on  PortDimensions=1
  Subsystem : Subsystem
  out : Outport
  wires:
  in/1 -> Subsystem/1(in)
  Subsystem/1(out) -> out/1
  Trigger/1 -> Subsystem/Enable

== system actuator_control/Contact Velocities/Velocity on Contact3 ==
  in : Inport
  Trigger : TriggerPort  ShowOutputPort=on  PortDimensions=1
  Subsystem : Subsystem
  out : Outport
  wires:
  Trigger/1 -> Subsystem/Enable
  Subsystem/1(out) -> out/1
  in/1 -> Subsystem/1(in)

== system actuator_control/SEA Controller (Velocity)/Integrator ==
  Signal : Inport
  Reset [1/0] : Inport  Port=2
  Demux : Demux
  Demux1 : Demux
  Discrete-Time Integrator{,1..3} (4 alike) : DiscreteIntegrator  ExternalReset=rising  InitialConditionSetting=State (most efficient)  SampleTime=sample_time  LimitOutput=on  UpperSaturationLimit=1  LowerSaturationLimit=-1
  Mux : Mux
  Integrated : Outport
  wires:
  Signal/1 -> Demux/1
  Discrete-Time Integrator/1 -> Mux/1
  Reset [1/0]/1 -> Demux1/1
  Mux/1 -> Integrated/1
  Discrete-Time Integrator1/1 -> Mux/2
  Discrete-Time Integrator2/1 -> Mux/3
  Discrete-Time Integrator3/1 -> Mux/4
  Demux1/4 -> Discrete-Time Integrator3/2
  Demux1/3 -> Discrete-Time Integrator2/2
  Demux1/2 -> Discrete-Time Integrator1/2
  Demux1/1 -> Discrete-Time Integrator/2
  Demux/1 -> Discrete-Time Integrator/1
  Demux/2 -> Discrete-Time Integrator1/1
  Demux/3 -> Discrete-Time Integrator2/1
  Demux/4 -> Discrete-Time Integrator3/1

== system actuator_control/SEA Controller (Velocity)/Lowpass Filter (Stance) ==
  In : Inport
  Generated Filter Block : DiscreteFir  Tag=BlockMethodSubSystem  Coefficients=[-0.049792265798371309 -0.00478204397482343 -0.0023545966524627579 0.0019617877955006649 0.0081617445920188422 0.01606136498204886 0.025426522925330174 0.035808512742994333 0.046780148761454213 0.057713212050140641 0.068077289761393753 0.077169075575072327 0.084565882051693325 0.089692876147162801 0.092473878579640248 0.092473878579640248 0.089692876147162801 0.084565882051693325 0.077169075575072327 0.068077289761393753 0.057713212050140641 0.046780148761454213 0.035808512742994333 0.025426522925330174 0.01606136498204886 0.0081617445920188422 0.0019617877955006649 -0.0023545966524627579 -0.00478204397482343 -0.049792265798371309]
  Out : Outport
  wires:
  In/1 -> Generated Filter Block/1
  Generated Filter Block/1 -> Out/1

== system actuator_control/SEA Controller (Velocity)/Lowpass Filter (Swing) ==
  In : Inport
  Generated Filter Block : dsparch4/Biquad Filter  Tag=BlockMethodSubSystem  IIRFiltStruct=Direct form II  CoeffSource=Specify via dialog  BiQuadCoeffs=[1.0218648663828083 -2 1.0218648663828083 1 -1.9114378222117407 0.91557643487411833]  a0Flag=Warning  IC=0  ICnum=0  ICden=0  denAccumFracLength=30  denProdOutputFracLength=30  secondMemoryFracLength=15  roundingMode=Floor  overflowMode=off  ScaleValues=[0.0041174265739107223;22.985401576126357]  optimizeScaleValues=off  ScaleValueMode=Specify via input port (g)  scaleValueFracLength=14  FilterSource=Specify via dialog  FilterObject=Hm_biquad
  Out : Outport
  wires:
  Generated Filter Block/1 -> Out/1
  In/1 -> Generated Filter Block/1

== system actuator_control/SEA Controller (Velocity)/Stance or Swing ==
  True/False x4 : Inport
  Signal True x4 : Inport  Port=2
  Signal False x4 : Inport  Port=3
  Demux : Demux
  Demux1 : Demux
  Demux2 : Demux
  Mux : Mux
  Switch{,1..3} (4 alike) : Switch  Criteria=u2 ~= 0
  Selected x4 : Outport
  wires:
  Mux/1 -> Selected x4/1
  True/False x4/1 -> Demux1/1
  Signal True x4/1 -> Demux/1
  Signal False x4/1 -> Demux2/1
  Demux/1 -> Switch/1
  Demux/2 -> Switch1/1
  Demux/3 -> Switch2/1
  Demux/4 -> Switch3/1
  Demux2/1 -> Switch/3
  Demux2/2 -> Switch1/3
  Demux2/3 -> Switch2/3
  Demux2/4 -> Switch3/3
  Demux1/1 -> Switch/2
  Demux1/2 -> Switch1/2
  Demux1/3 -> Switch2/2
  Demux1/4 -> Switch3/2
  Switch/1 -> Mux/1
  Switch1/1 -> Mux/2
  Switch2/1 -> Mux/3
  Switch3/1 -> Mux/4

== system actuator_control/SEA Controller (Velocity)/Stance or Swing1 ==
  True/False x4 : Inport
  Signal True x4 : Inport  Port=2
  Signal False x4 : Inport  Port=3
  Demux : Demux
  Demux1 : Demux
  Demux2 : Demux
  Mux : Mux
  Switch{,1..3} (4 alike) : Switch  Criteria=u2 ~= 0
  Selected x4 : Outport
  wires:
  Switch3/1 -> Mux/4
  Switch2/1 -> Mux/3
  Switch1/1 -> Mux/2
  Switch/1 -> Mux/1
  Demux1/4 -> Switch3/2
  Demux1/3 -> Switch2/2
  Demux1/2 -> Switch1/2
  Demux1/1 -> Switch/2
  Demux2/4 -> Switch3/3
  Demux2/3 -> Switch2/3
  Demux2/2 -> Switch1/3
  Demux2/1 -> Switch/3
  Demux/4 -> Switch3/1
  Demux/3 -> Switch2/1
  Demux/2 -> Switch1/1
  Demux/1 -> Switch/1
  Signal False x4/1 -> Demux2/1
  Signal True x4/1 -> Demux/1
  True/False x4/1 -> Demux1/1
  Mux/1 -> Selected x4/1

== system actuator_control/SEA Controller (Velocity)/Stance or Swing2 ==
  True/False x4 : Inport
  Signal True x4 : Inport  Port=2
  Signal False x4 : Inport  Port=3
  Demux : Demux
  Demux1 : Demux
  Demux2 : Demux
  Mux : Mux
  Switch{,1..3} (4 alike) : Switch  Criteria=u2 ~= 0
  Selected x4 : Outport
  wires:
  Mux/1 -> Selected x4/1
  True/False x4/1 -> Demux1/1
  Signal True x4/1 -> Demux/1
  Signal False x4/1 -> Demux2/1
  Demux/1 -> Switch/1
  Demux/2 -> Switch1/1
  Demux/3 -> Switch2/1
  Demux/4 -> Switch3/1
  Demux2/1 -> Switch/3
  Demux2/2 -> Switch1/3
  Demux2/3 -> Switch2/3
  Demux2/4 -> Switch3/3
  Demux1/1 -> Switch/2
  Demux1/2 -> Switch1/2
  Demux1/3 -> Switch2/2
  Demux1/4 -> Switch3/2
  Switch/1 -> Mux/1
  Switch1/1 -> Mux/2
  Switch2/1 -> Mux/3
  Switch3/1 -> Mux/4

== system actuator_control/Timers/Time on Contact ==
  in : Inport
  Trigger : TriggerPort  ShowOutputPort=on  PortDimensions=1
  Subsystem : Subsystem
  out : Outport
  wires:
  in/1 -> Subsystem/1(in)
  Subsystem/1(out) -> out/1
  Trigger/1 -> Subsystem/Enable

== system actuator_control/Timers/Time on Contact1 ==
  in : Inport
  Trigger : TriggerPort  ShowOutputPort=on  PortDimensions=1
  Subsystem : Subsystem
  out : Outport
  wires:
  Trigger/1 -> Subsystem/Enable
  Subsystem/1(out) -> out/1
  in/1 -> Subsystem/1(in)

== system actuator_control/Timers/Time on Contact2 ==
  in : Inport
  Trigger : TriggerPort  ShowOutputPort=on  PortDimensions=1
  Subsystem : Subsystem
  out : Outport
  wires:
  Trigger/1 -> Subsystem/Enable
  Subsystem/1(out) -> out/1
  in/1 -> Subsystem/1(in)

== system actuator_control/Timers/Time on Contact3 ==
  in : Inport
  Trigger : TriggerPort  ShowOutputPort=on  PortDimensions=1
  Subsystem : Subsystem
  out : Outport
  wires:
  in/1 -> Subsystem/1(in)
  Subsystem/1(out) -> out/1
  Trigger/1 -> Subsystem/Enable

== system actuator_control/Contact Velocities/Velocity on Contact/Subsystem ==
  in : Inport
  Enable : EnablePort
  out : Outport
  wires:
  in/1 -> out/1

== system actuator_control/Contact Velocities/Velocity on Contact1/Subsystem ==
  in : Inport
  Enable : EnablePort
  out : Outport
  wires:
  in/1 -> out/1

== system actuator_control/Contact Velocities/Velocity on Contact2/Subsystem ==
  in : Inport
  Enable : EnablePort
  out : Outport
  wires:
  in/1 -> out/1

== system actuator_control/Contact Velocities/Velocity on Contact3/Subsystem ==
  in : Inport
  Enable : EnablePort
  out : Outport
  wires:
  in/1 -> out/1

== system actuator_control/Timers/Time on Contact/Subsystem ==
  in : Inport
  Enable : EnablePort
  out : Outport
  wires:
  in/1 -> out/1

== system actuator_control/Timers/Time on Contact1/Subsystem ==
  in : Inport
  Enable : EnablePort
  out : Outport
  wires:
  in/1 -> out/1

== system actuator_control/Timers/Time on Contact2/Subsystem ==
  in : Inport
  Enable : EnablePort
  out : Outport
  wires:
  in/1 -> out/1

== system actuator_control/Timers/Time on Contact3/Subsystem ==
  in : Inport
  Enable : EnablePort
  out : Outport
  wires:
  in/1 -> out/1
